simulink model "smP6"  (R2023b)
settings: Solver=VariableStepAuto  StartTime=0.0  StopTime=0.005  FixedStep=1e-10  RelTol=1e-3
model workspace (MAT data in the model file):
  C = 1e-05
  L = 0.002
  R = 10
settings Model: Creator=mluser  LastModifiedBy=mluser

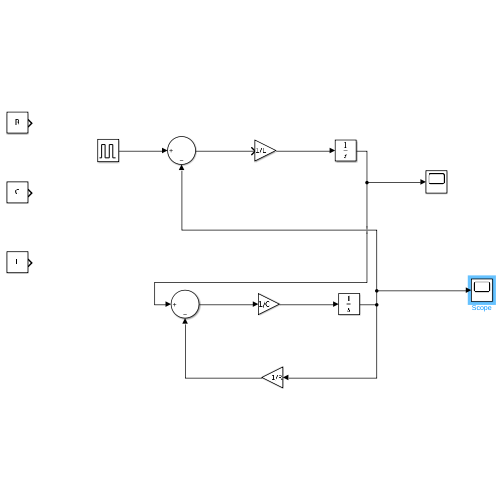
[thumbnail: Simulink's stored preview of the top-level diagram]
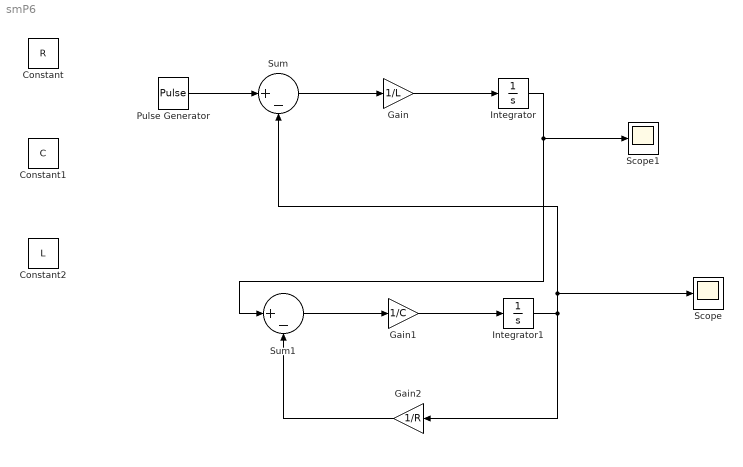
== system smP6 ==
  Constant : Constant  Value=R
  Constant1 : Constant  Value=C
  Constant2 : Constant  Value=L
  Gain : Gain  Gain=1/L
  Gain1 : Gain  Gain=1/C
  Gain2 : Gain  Gain=1/R
  Integrator : Integrator
  Integrator1 : Integrator
  Pulse Generator : DiscretePulseGenerator  PulseType=Time based  Amplitude=32  Period=(1e-5)  PulseWidth=38
  Scope : Scope
  Scope1 : Scope
  Sum : Sum  Inputs=|+-
  Sum1 : Sum  Inputs=|+-
  wires:
  Gain/1 -> Integrator/1
  Gain1/1 -> Integrator1/1
  Sum/1 -> Gain/1
  Integrator1/1 -> Gain2/1, Scope/1, Sum/2
  Sum1/1 -> Gain1/1
  Gain2/1 -> Sum1/2
  Integrator/1 -> Scope1/1, Sum1/1
  Pulse Generator/1 -> Sum/1
